simulink model "statespace"  (R2021a)
settings: Solver=FixedStepAuto  StartTime=0.0  StopTime=inf  FixedStep=Ts  RelTol=1e-3
values from neighbouring files (symbols this model uses):
  Kt = 0.882355004501468    (= 0.882355004501)    [initModels_GUI.m]
undefined symbols (not defined in the file or in its folder): Tqe_Aft, Tqe_Bow
libraries: slident x2
settings Model: Creator=EGI-Z400  LastModifiedBy=EGI-Z400
settings SolverCC: ConcurrentTasks=on  PositivePriorityOrder=on
settings OptimizationCC: BlockReduction=off  OptimizeBlockIOStorage=off
settings DebuggingCC: TasksWithSamePriorityMsg=none
settings HardwareCC: ProdBitPerLong=64  ProdLongLongMode=on  ProdHWDeviceType=Intel->x86-64 (Linux 64)
settings RTWCC: Description=Simulink Real-Time  SystemTargetFile=slrealtime.tlc  TemplateMakefile=slrealtime_default_tmf  Toolchain=Simulink Real-Time Toolchain  BuildConfiguration=Faster Runs  CodeExecutionProfiling=on  TargetLang=C++

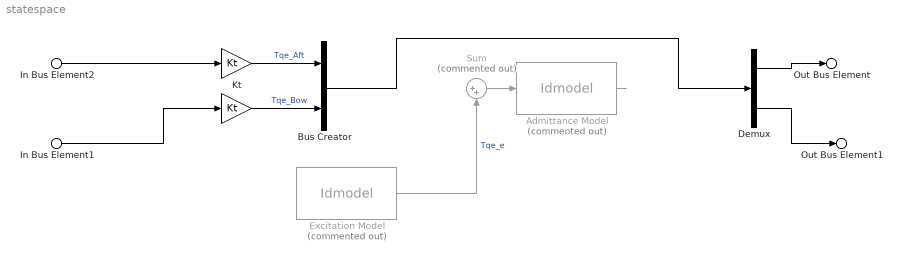
== system statespace ==
  In Bus Element1 : Inport  PortName=ctrl2twin  Element=Cur_Bow
  In Bus Element2 : Inport  PortName=ctrl2twin  Element=Cur_Aft
  " " : Gain  Gain=Kt
  Admittance Model : slident/Models/Idmodel  Commented=on  sys=admittance  IC=0  noi=off  seed=[]
      settings: SourceProductBaseCode=ID
  Bus Creator : BusCreator  Inputs=Tqe_Aft,Tqe_Bow  OutDataTypeStr=Bus: torqueBus
  Demux : Demux  Outputs=2
  Excitation Model : slident/Models/Idmodel  Commented=on  sys=excitation  IC=0  noi=off  seed=[]
      settings: SourceProductBaseCode=ID
  Kt : Gain  Gain=Kt
  Sum : Sum  Commented=on  Inputs=|++
  Out Bus Element : Outport  PortName=twin2ctrl  Element=Pos_Aft
  Out Bus Element1 : Outport  PortName=twin2ctrl  Element=Pos_Bow
  wires:
  Admittance Model/1 -> ?
  In Bus Element1/1 -> " "/1
  Demux/2 -> Out Bus Element1/1
  Kt/1 -> Bus Creator/1  "Tqe_Aft"
  Sum/1 -> Admittance Model/1
  In Bus Element2/1 -> Kt/1
  Demux/1 -> Out Bus Element/1
  " "/1 -> Bus Creator/2  "Tqe_Bow"
  Excitation Model/1 -> Sum/2  "Tqe_e"
  Bus Creator/1 -> Demux/1
